simulink model "HybridBus_BEVModel"  (R2025a)
settings: Solver=FixedStepDiscrete  StartTime=0.0  StopTime=Input.Route.Time_s(end)  FixedStep=model_sample_time_s  RelTol=1e-3
InitFcn:
  | assign_hybrid_bus_model_workspace;
undefined symbols (not defined in the file): air_density_kg_m3, auxiliary_base_power_kw, auxiliary_override, battery1_charge_efficiency, battery1_discharge_efficiency, battery1_initial_energy_kwh, battery1_max_charge_kw, battery1_max_discharge_kw, battery1_max_energy_kwh, battery1_min_energy_kwh, battery1_usable_energy_kwh, battery2_charge_efficiency, battery2_discharge_efficiency, battery2_initial_energy_kwh, battery2_max_charge_kw, battery2_max_discharge_kw, battery2_max_energy_kwh, battery2_min_energy_kwh, battery2_usable_energy_kwh, BEVUseTwoBatteries, DiscIntNeverNeededParam, drag_coefficient, electricity_price_per_kWh, final_drive_motoring_efficiency, final_drive_ratio, final_drive_regen_efficiency, frontal_area_m2, fuel_price_per_L, gravity_m_s2, grid_charge_efficiency, model_sample_time_s, motor_max_speed_rpm, motor_motoring_efficiency, motor_regen_efficiency, motor_regen_limit_kw, motor_traction_limit_kw, rolling_coefficient, tyre_radius_m, vehicle_mass_kg
settings Model: Creator=Karuna  LastModifiedBy=Karuna
settings DataIOCC: SaveOutput=off  SignalLogging=off

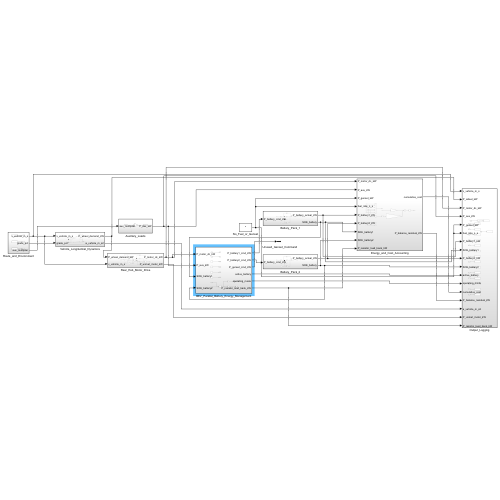
[thumbnail: Simulink's stored preview of the top-level diagram]
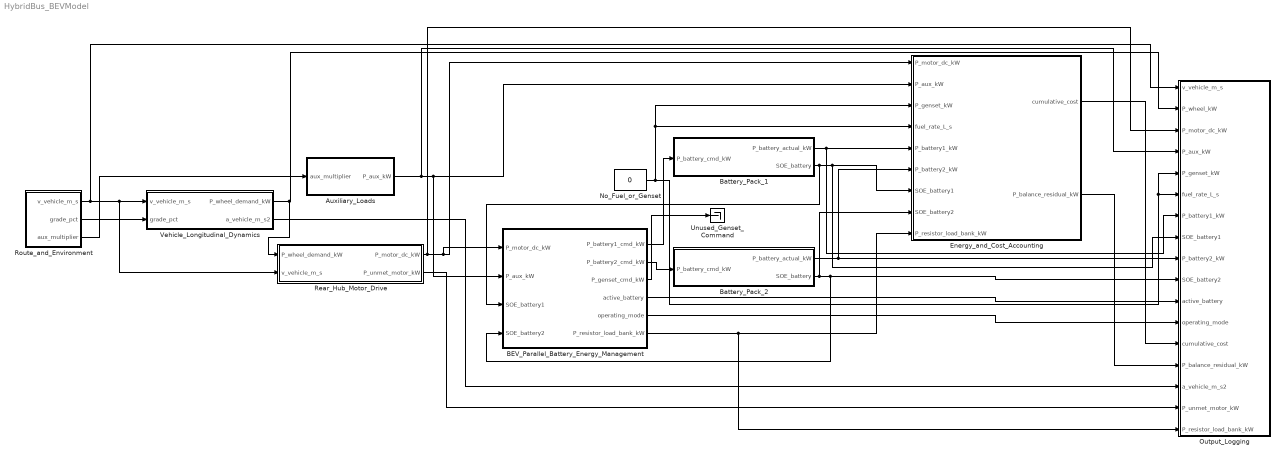
== system HybridBus_BEVModel ==
  Auxiliary_Loads : Subsystem
  BEV_Parallel_Battery_Energy_Management : Subsystem
  Battery_Pack_1 : Subsystem
  Battery_Pack_2 : Subsystem
  Energy_and_Cost_Accounting : Subsystem
  No_Fuel_or_Genset : Constant  Value=0
  Output_Logging : Subsystem
  Rear_Hub_Motor_Drive : Subsystem
  Route_and_Environment : Subsystem
  Unused_Genset_Command : Terminator
  Vehicle_Longitudinal_Dynamics : Subsystem
  wires:
  Route_and_Environment/2(grade_pct) -> Vehicle_Longitudinal_Dynamics/2(grade_pct)
  No_Fuel_or_Genset/1 -> Output_Logging/6(fuel_rate_L_s), Output_Logging/5(P_genset_kW), Energy_and_Cost_Accounting/4(fuel_rate_L_s), Energy_and_Cost_Accounting/3(P_genset_kW)
  Energy_and_Cost_Accounting/2(P_balance_residual_kW) -> Output_Logging/14(P_balance_residual_kW)
  Energy_and_Cost_Accounting/1(cumulative_cost) -> Output_Logging/13(cumulative_cost)
  Battery_Pack_2/1(P_battery_actual_kW) -> Energy_and_Cost_Accounting/6(P_battery2_kW), Output_Logging/9(P_battery2_kW)
  Battery_Pack_1/1(P_battery_actual_kW) -> Energy_and_Cost_Accounting/5(P_battery1_kW), Output_Logging/7(P_battery1_kW)
  Rear_Hub_Motor_Drive/2(P_unmet_motor_kW) -> Output_Logging/16(P_unmet_motor_kW)
  Vehicle_Longitudinal_Dynamics/2(a_vehicle_m_s2) -> Output_Logging/15(a_vehicle_m_s2)
  Vehicle_Longitudinal_Dynamics/1(P_wheel_demand_kW) -> Output_Logging/2(P_wheel_kW), Rear_Hub_Motor_Drive/1(P_wheel_demand_kW)
  Route_and_Environment/1(v_vehicle_m_s) -> Vehicle_Longitudinal_Dynamics/1(v_vehicle_m_s), Rear_Hub_Motor_Drive/2(v_vehicle_m_s), Output_Logging/1(v_vehicle_m_s)
  Route_and_Environment/3(aux_multiplier) -> Auxiliary_Loads/1(aux_multiplier)
  BEV_Parallel_Battery_Energy_Management/3(P_genset_cmd_kW) -> Unused_Genset_Command/1
  Battery_Pack_2/2(SOE_battery) -> Output_Logging/10(SOE_battery2), BEV_Parallel_Battery_Energy_Management/4(SOE_battery2), Energy_and_Cost_Accounting/8(SOE_battery2)
  Auxiliary_Loads/1(P_aux_kW) -> Energy_and_Cost_Accounting/2(P_aux_kW), BEV_Parallel_Battery_Energy_Management/2(P_aux_kW), Output_Logging/4(P_aux_kW)
  Rear_Hub_Motor_Drive/1(P_motor_dc_kW) -> Energy_and_Cost_Accounting/1(P_motor_dc_kW), BEV_Parallel_Battery_Energy_Management/1(P_motor_dc_kW), Output_Logging/3(P_motor_dc_kW)
  Battery_Pack_1/2(SOE_battery) -> Energy_and_Cost_Accounting/7(SOE_battery1), Output_Logging/8(SOE_battery1), BEV_Parallel_Battery_Energy_Management/3(SOE_battery1)
  BEV_Parallel_Battery_Energy_Management/1(P_battery1_cmd_kW) -> Battery_Pack_1/1(P_battery_cmd_kW)
  BEV_Parallel_Battery_Energy_Management/2(P_battery2_cmd_kW) -> Battery_Pack_2/1(P_battery_cmd_kW)
  BEV_Parallel_Battery_Energy_Management/4(active_battery) -> Output_Logging/11(active_battery)
  BEV_Parallel_Battery_Energy_Management/5(operating_mode) -> Output_Logging/12(operating_mode)
  BEV_Parallel_Battery_Energy_Management/6(P_resistor_load_bank_kW) -> Energy_and_Cost_Accounting/9(P_resistor_load_bank_kW), Output_Logging/17(P_resistor_load_bank_kW)

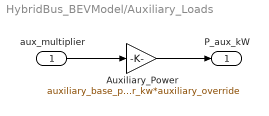
== system HybridBus_BEVModel/Auxiliary_Loads ==
  aux_multiplier : Inport
  Auxiliary_Power : Gain  Gain=auxiliary_base_power_kw*auxiliary_override
  P_aux_kW : Outport
  wires:
  Auxiliary_Power/1 -> P_aux_kW/1
  aux_multiplier/1 -> Auxiliary_Power/1

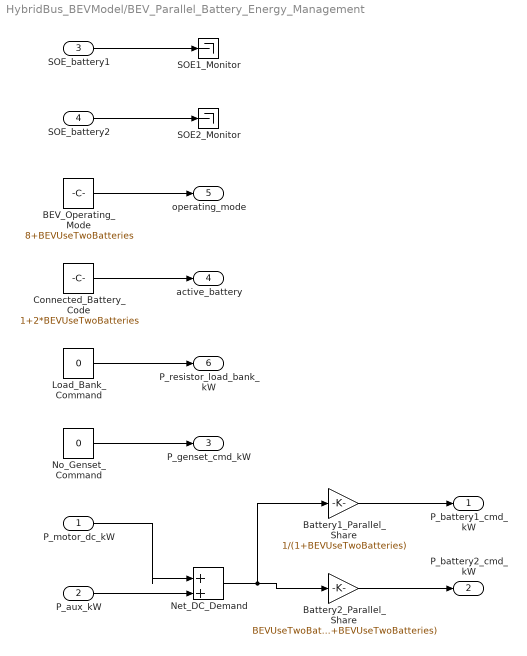
== system HybridBus_BEVModel/BEV_Parallel_Battery_Energy_Management ==
  P_motor_dc_kW : Inport
  P_aux_kW : Inport  Port=2
  SOE_battery1 : Inport  Port=3
  SOE_battery2 : Inport  Port=4
  BEV_Operating_Mode : Constant  Value=8+BEVUseTwoBatteries
  Battery1_Parallel_Share : Gain  Gain=1/(1+BEVUseTwoBatteries)
  Battery2_Parallel_Share : Gain  Gain=BEVUseTwoBatteries/(1+BEVUseTwoBatteries)
  Connected_Battery_Code : Constant  Value=1+2*BEVUseTwoBatteries
  Load_Bank_Command : Constant  Value=0
  Net_DC_Demand : Sum  Inputs=|++
  No_Genset_Command : Constant  Value=0
  SOE1_Monitor : Terminator
  SOE2_Monitor : Terminator
  P_battery1_cmd_kW : Outport
  P_battery2_cmd_kW : Outport  Port=2
  P_genset_cmd_kW : Outport  Port=3
  active_battery : Outport  Port=4
  operating_mode : Outport  Port=5
  P_resistor_load_bank_kW : Outport  Port=6
  wires:
  SOE_battery2/1 -> SOE2_Monitor/1
  SOE_battery1/1 -> SOE1_Monitor/1
  Load_Bank_Command/1 -> P_resistor_load_bank_kW/1
  BEV_Operating_Mode/1 -> operating_mode/1
  Connected_Battery_Code/1 -> active_battery/1
  No_Genset_Command/1 -> P_genset_cmd_kW/1
  Battery2_Parallel_Share/1 -> P_battery2_cmd_kW/1
  Battery1_Parallel_Share/1 -> P_battery1_cmd_kW/1
  Net_DC_Demand/1 -> Battery1_Parallel_Share/1, Battery2_Parallel_Share/1
  P_aux_kW/1 -> Net_DC_Demand/2
  P_motor_dc_kW/1 -> Net_DC_Demand/1

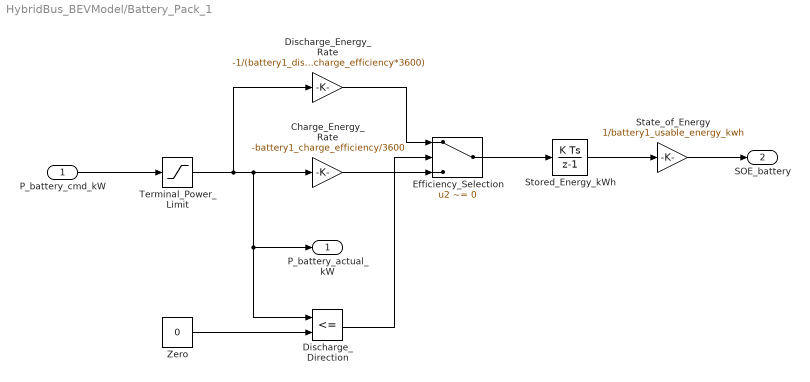
== system HybridBus_BEVModel/Battery_Pack_1 ==
  P_battery_cmd_kW : Inport
  Charge_Energy_Rate : Gain  Gain=-battery1_charge_efficiency/3600
  Discharge_Direction : RelationalOperator  Operator=<=  OutDataTypeStr=boolean  RndMeth=Simplest  InputSameDT=off
  Discharge_Energy_Rate : Gain  Gain=-1/(battery1_discharge_efficiency*3600)
  Efficiency_Selection : Switch  Criteria=u2 ~= 0  SaturateOnIntegerOverflow=off  InputSameDT=off
  State_of_Energy : Gain  Gain=1/battery1_usable_energy_kwh
  Stored_Energy_kWh : DiscreteIntegrator  InitialCondition=battery1_initial_energy_kwh  SampleTime=model_sample_time_s  LimitOutput=on  UpperSaturationLimit=battery1_max_energy_kwh  LowerSaturationLimit=battery1_min_energy_kwh  ICPrevOutput=DiscIntNeverNeededParam  ICPrevScaledInput=DiscIntNeverNeededParam
  Terminal_Power_Limit : Saturate  UpperLimit=battery1_max_discharge_kw  LowerLimit=-battery1_max_charge_kw
  Zero : Constant  Value=0
  P_battery_actual_kW : Outport
  SOE_battery : Outport  Port=2
  wires:
  State_of_Energy/1 -> SOE_battery/1
  Stored_Energy_kWh/1 -> State_of_Energy/1
  Efficiency_Selection/1 -> Stored_Energy_kWh/1
  Charge_Energy_Rate/1 -> Efficiency_Selection/3
  Discharge_Direction/1 -> Efficiency_Selection/2
  Discharge_Energy_Rate/1 -> Efficiency_Selection/1
  Zero/1 -> Discharge_Direction/2
  Terminal_Power_Limit/1 -> P_battery_actual_kW/1, Discharge_Direction/1, Charge_Energy_Rate/1, Discharge_Energy_Rate/1
  P_battery_cmd_kW/1 -> Terminal_Power_Limit/1

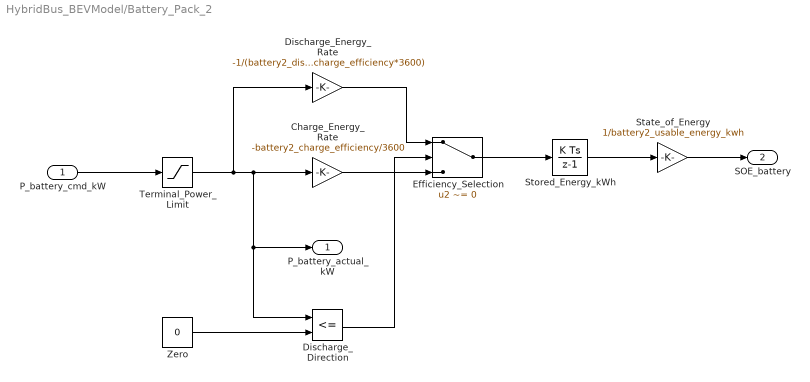
== system HybridBus_BEVModel/Battery_Pack_2 ==
  P_battery_cmd_kW : Inport
  Charge_Energy_Rate : Gain  Gain=-battery2_charge_efficiency/3600
  Discharge_Direction : RelationalOperator  Operator=<=  OutDataTypeStr=boolean  RndMeth=Simplest  InputSameDT=off
  Discharge_Energy_Rate : Gain  Gain=-1/(battery2_discharge_efficiency*3600)
  Efficiency_Selection : Switch  Criteria=u2 ~= 0  SaturateOnIntegerOverflow=off  InputSameDT=off
  State_of_Energy : Gain  Gain=1/battery2_usable_energy_kwh
  Stored_Energy_kWh : DiscreteIntegrator  InitialCondition=battery2_initial_energy_kwh  SampleTime=model_sample_time_s  LimitOutput=on  UpperSaturationLimit=battery2_max_energy_kwh  LowerSaturationLimit=battery2_min_energy_kwh  ICPrevOutput=DiscIntNeverNeededParam  ICPrevScaledInput=DiscIntNeverNeededParam
  Terminal_Power_Limit : Saturate  UpperLimit=battery2_max_discharge_kw  LowerLimit=-battery2_max_charge_kw
  Zero : Constant  Value=0
  P_battery_actual_kW : Outport
  SOE_battery : Outport  Port=2
  wires:
  State_of_Energy/1 -> SOE_battery/1
  Stored_Energy_kWh/1 -> State_of_Energy/1
  Efficiency_Selection/1 -> Stored_Energy_kWh/1
  Charge_Energy_Rate/1 -> Efficiency_Selection/3
  Discharge_Direction/1 -> Efficiency_Selection/2
  Discharge_Energy_Rate/1 -> Efficiency_Selection/1
  Zero/1 -> Discharge_Direction/2
  Terminal_Power_Limit/1 -> P_battery_actual_kW/1, Discharge_Direction/1, Charge_Energy_Rate/1, Discharge_Energy_Rate/1
  P_battery_cmd_kW/1 -> Terminal_Power_Limit/1

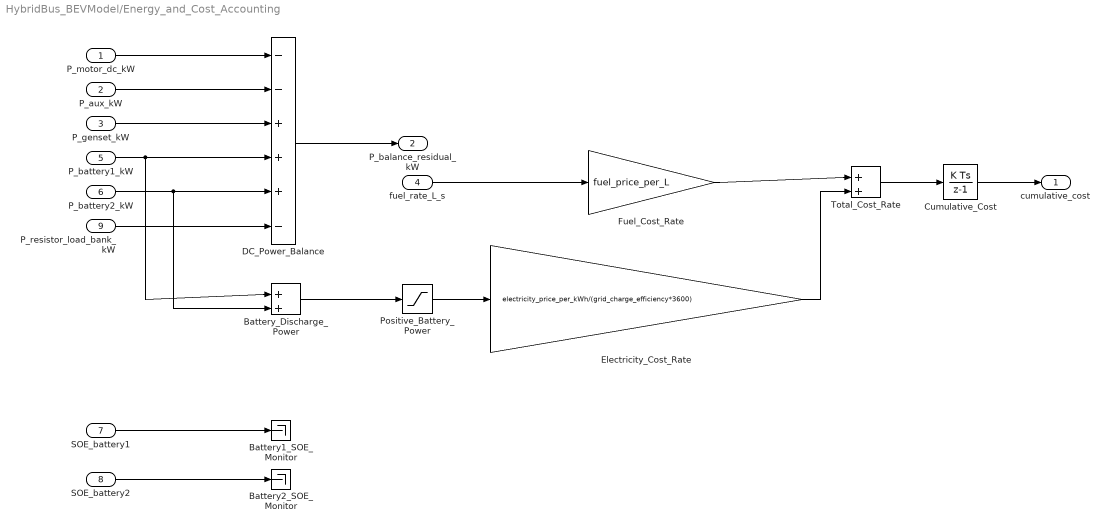
== system HybridBus_BEVModel/Energy_and_Cost_Accounting ==
  P_motor_dc_kW : Inport
  P_aux_kW : Inport  Port=2
  P_genset_kW : Inport  Port=3
  fuel_rate_L_s : Inport  Port=4
  P_battery1_kW : Inport  Port=5
  P_battery2_kW : Inport  Port=6
  SOE_battery1 : Inport  Port=7
  SOE_battery2 : Inport  Port=8
  P_resistor_load_bank_kW : Inport  Port=9
  Battery1_SOE_Monitor : Terminator
  Battery2_SOE_Monitor : Terminator
  Battery_Discharge_Power : Sum  Inputs=|++
  Cumulative_Cost : DiscreteIntegrator  SampleTime=model_sample_time_s  ICPrevOutput=DiscIntNeverNeededParam  ICPrevScaledInput=DiscIntNeverNeededParam
  DC_Power_Balance : Sum  Inputs=--+++-
  Electricity_Cost_Rate : Gain  Gain=electricity_price_per_kWh/(grid_charge_efficiency*3600)
  Fuel_Cost_Rate : Gain  Gain=fuel_price_per_L
  Positive_Battery_Power : Saturate  UpperLimit=inf  LowerLimit=0
  Total_Cost_Rate : Sum  Inputs=|++
  cumulative_cost : Outport
  P_balance_residual_kW : Outport  Port=2
  wires:
  fuel_rate_L_s/1 -> Fuel_Cost_Rate/1
  P_aux_kW/1 -> DC_Power_Balance/2
  P_battery2_kW/1 -> Battery_Discharge_Power/2, DC_Power_Balance/5
  P_motor_dc_kW/1 -> DC_Power_Balance/1
  P_genset_kW/1 -> DC_Power_Balance/3
  P_battery1_kW/1 -> Battery_Discharge_Power/1, DC_Power_Balance/4
  SOE_battery2/1 -> Battery2_SOE_Monitor/1
  Battery_Discharge_Power/1 -> Positive_Battery_Power/1
  P_resistor_load_bank_kW/1 -> DC_Power_Balance/6
  SOE_battery1/1 -> Battery1_SOE_Monitor/1
  Cumulative_Cost/1 -> cumulative_cost/1
  DC_Power_Balance/1 -> P_balance_residual_kW/1
  Total_Cost_Rate/1 -> Cumulative_Cost/1
  Positive_Battery_Power/1 -> Electricity_Cost_Rate/1
  Fuel_Cost_Rate/1 -> Total_Cost_Rate/1
  Electricity_Cost_Rate/1 -> Total_Cost_Rate/2

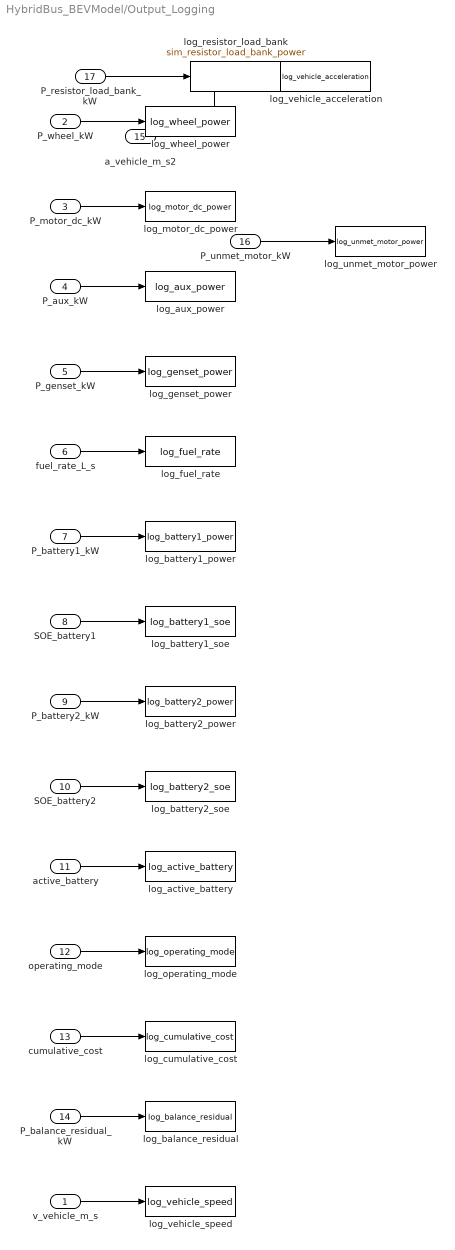
== system HybridBus_BEVModel/Output_Logging ==
  v_vehicle_m_s : Inport
  P_wheel_kW : Inport  Port=2
  P_motor_dc_kW : Inport  Port=3
  P_aux_kW : Inport  Port=4
  P_genset_kW : Inport  Port=5
  fuel_rate_L_s : Inport  Port=6
  P_battery1_kW : Inport  Port=7
  SOE_battery1 : Inport  Port=8
  P_battery2_kW : Inport  Port=9
  SOE_battery2 : Inport  Port=10
  active_battery : Inport  Port=11
  operating_mode : Inport  Port=12
  cumulative_cost : Inport  Port=13
  P_balance_residual_kW : Inport  Port=14
  a_vehicle_m_s2 : Inport  Port=15
  P_unmet_motor_kW : Inport  Port=16
  P_resistor_load_bank_kW : Inport  Port=17
  log_active_battery : ToWorkspace  VariableName=log_active_battery  SaveFormat=Timeseries  SampleTime=-1
  log_aux_power : ToWorkspace  VariableName=log_aux_power  SaveFormat=Timeseries  SampleTime=-1
  log_balance_residual : ToWorkspace  VariableName=log_balance_residual  SaveFormat=Timeseries  SampleTime=-1
  log_battery1_power : ToWorkspace  VariableName=log_battery1_power  SaveFormat=Timeseries  SampleTime=-1
  log_battery1_soe : ToWorkspace  VariableName=log_battery1_soe  SaveFormat=Timeseries  SampleTime=-1
  log_battery2_power : ToWorkspace  VariableName=log_battery2_power  SaveFormat=Timeseries  SampleTime=-1
  log_battery2_soe : ToWorkspace  VariableName=log_battery2_soe  SaveFormat=Timeseries  SampleTime=-1
  log_cumulative_cost : ToWorkspace  VariableName=log_cumulative_cost  SaveFormat=Timeseries  SampleTime=-1
  log_fuel_rate : ToWorkspace  VariableName=log_fuel_rate  SaveFormat=Timeseries  SampleTime=-1
  log_genset_power : ToWorkspace  VariableName=log_genset_power  SaveFormat=Timeseries  SampleTime=-1
  log_motor_dc_power : ToWorkspace  VariableName=log_motor_dc_power  SaveFormat=Timeseries  SampleTime=-1
  log_operating_mode : ToWorkspace  VariableName=log_operating_mode  SaveFormat=Timeseries  SampleTime=-1
  log_resistor_load_bank : ToWorkspace  VariableName=sim_resistor_load_bank_power  SampleTime=-1
  log_unmet_motor_power : ToWorkspace  VariableName=log_unmet_motor_power  SaveFormat=Timeseries  SampleTime=-1
  log_vehicle_acceleration : ToWorkspace  VariableName=log_vehicle_acceleration  SaveFormat=Timeseries  SampleTime=-1
  log_vehicle_speed : ToWorkspace  VariableName=log_vehicle_speed  SaveFormat=Timeseries  SampleTime=-1
  log_wheel_power : ToWorkspace  VariableName=log_wheel_power  SaveFormat=Timeseries  SampleTime=-1
  wires:
  P_balance_residual_kW/1 -> log_balance_residual/1
  cumulative_cost/1 -> log_cumulative_cost/1
  operating_mode/1 -> log_operating_mode/1
  active_battery/1 -> log_active_battery/1
  SOE_battery2/1 -> log_battery2_soe/1
  P_battery2_kW/1 -> log_battery2_power/1
  SOE_battery1/1 -> log_battery1_soe/1
  P_battery1_kW/1 -> log_battery1_power/1
  fuel_rate_L_s/1 -> log_fuel_rate/1
  P_genset_kW/1 -> log_genset_power/1
  P_aux_kW/1 -> log_aux_power/1
  P_motor_dc_kW/1 -> log_motor_dc_power/1
  P_wheel_kW/1 -> log_wheel_power/1
  v_vehicle_m_s/1 -> log_vehicle_speed/1
  P_unmet_motor_kW/1 -> log_unmet_motor_power/1
  P_resistor_load_bank_kW/1 -> log_resistor_load_bank/1
  a_vehicle_m_s2/1 -> log_vehicle_acceleration/1

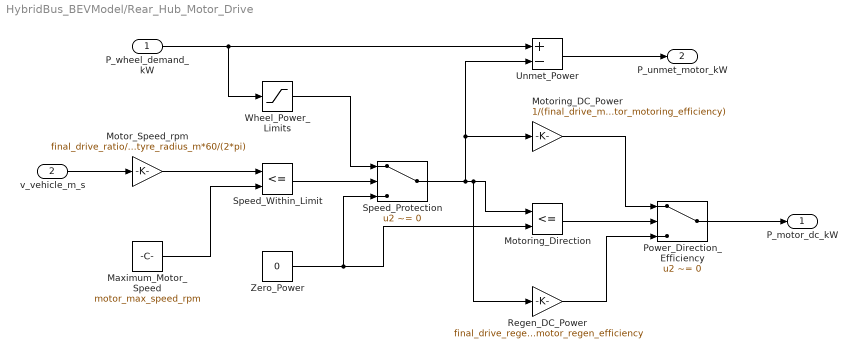
== system HybridBus_BEVModel/Rear_Hub_Motor_Drive ==
  P_wheel_demand_kW : Inport
  v_vehicle_m_s : Inport  Port=2
  Maximum_Motor_Speed : Constant  Value=motor_max_speed_rpm
  Motor_Speed_rpm : Gain  Gain=final_drive_ratio/tyre_radius_m*60/(2*pi)
  Motoring_DC_Power : Gain  Gain=1/(final_drive_motoring_efficiency*motor_motoring_efficiency)
  Motoring_Direction : RelationalOperator  Operator=<=  OutDataTypeStr=boolean  RndMeth=Simplest  InputSameDT=off
  Power_Direction_Efficiency : Switch  Criteria=u2 ~= 0  SaturateOnIntegerOverflow=off  InputSameDT=off
  Regen_DC_Power : Gain  Gain=final_drive_regen_efficiency*motor_regen_efficiency
  Speed_Protection : Switch  Criteria=u2 ~= 0  SaturateOnIntegerOverflow=off  InputSameDT=off
  Speed_Within_Limit : RelationalOperator  Operator=<=  OutDataTypeStr=boolean  RndMeth=Simplest  InputSameDT=off
  Unmet_Power : Sum  Inputs=+-
  Wheel_Power_Limits : Saturate  UpperLimit=motor_traction_limit_kw  LowerLimit=-motor_regen_limit_kw
  Zero_Power : Constant  Value=0
  P_motor_dc_kW : Outport
  P_unmet_motor_kW : Outport  Port=2
  wires:
  Unmet_Power/1 -> P_unmet_motor_kW/1
  Power_Direction_Efficiency/1 -> P_motor_dc_kW/1
  Regen_DC_Power/1 -> Power_Direction_Efficiency/3
  Motoring_Direction/1 -> Power_Direction_Efficiency/2
  Motoring_DC_Power/1 -> Power_Direction_Efficiency/1
  Speed_Protection/1 -> Regen_DC_Power/1, Motoring_Direction/1, Motoring_DC_Power/1, Unmet_Power/2
  Zero_Power/1 -> Speed_Protection/3, Motoring_Direction/2
  Speed_Within_Limit/1 -> Speed_Protection/2
  Wheel_Power_Limits/1 -> Speed_Protection/1
  Maximum_Motor_Speed/1 -> Speed_Within_Limit/2
  Motor_Speed_rpm/1 -> Speed_Within_Limit/1
  v_vehicle_m_s/1 -> Motor_Speed_rpm/1
  P_wheel_demand_kW/1 -> Unmet_Power/1, Wheel_Power_Limits/1

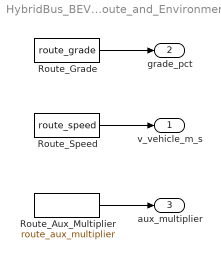
== system HybridBus_BEVModel/Route_and_Environment ==
  Route_Aux_Multiplier : FromWorkspace  VariableName=route_aux_multiplier
  Route_Grade : FromWorkspace  VariableName=route_grade
  Route_Speed : FromWorkspace  VariableName=route_speed
  v_vehicle_m_s : Outport
  grade_pct : Outport  Port=2
  aux_multiplier : Outport  Port=3
  wires:
  Route_Aux_Multiplier/1 -> aux_multiplier/1
  Route_Grade/1 -> grade_pct/1
  Route_Speed/1 -> v_vehicle_m_s/1

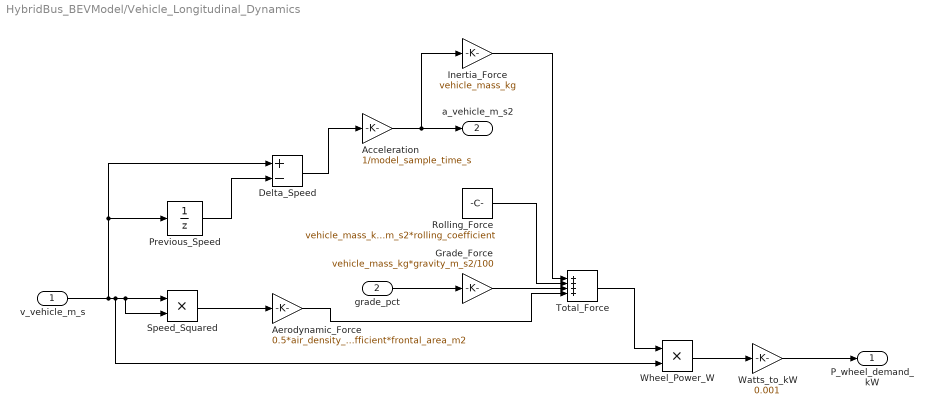
== system HybridBus_BEVModel/Vehicle_Longitudinal_Dynamics ==
  v_vehicle_m_s : Inport
  grade_pct : Inport  Port=2
  Acceleration : Gain  Gain=1/model_sample_time_s
  Aerodynamic_Force : Gain  Gain=0.5*air_density_kg_m3*drag_coefficient*frontal_area_m2
  Delta_Speed : Sum  Inputs=+-
  Grade_Force : Gain  Gain=vehicle_mass_kg*gravity_m_s2/100
  Inertia_Force : Gain  Gain=vehicle_mass_kg
  Previous_Speed : UnitDelay  SampleTime=model_sample_time_s  HasFrameUpgradeWarning=on
  Rolling_Force : Constant  Value=vehicle_mass_kg*gravity_m_s2*rolling_coefficient
  Speed_Squared : Product  Inputs=**
  Total_Force : Sum  Inputs=++++
  Watts_to_kW : Gain  Gain=0.001
  Wheel_Power_W : Product  Inputs=**
  P_wheel_demand_kW : Outport
  a_vehicle_m_s2 : Outport  Port=2
  wires:
  Watts_to_kW/1 -> P_wheel_demand_kW/1
  Wheel_Power_W/1 -> Watts_to_kW/1
  Total_Force/1 -> Wheel_Power_W/1
  Aerodynamic_Force/1 -> Total_Force/4
  Grade_Force/1 -> Total_Force/3
  Rolling_Force/1 -> Total_Force/2
  Inertia_Force/1 -> Total_Force/1
  Speed_Squared/1 -> Aerodynamic_Force/1
  grade_pct/1 -> Grade_Force/1
  Acceleration/1 -> a_vehicle_m_s2/1, Inertia_Force/1
  Delta_Speed/1 -> Acceleration/1
  Previous_Speed/1 -> Delta_Speed/2
  v_vehicle_m_s/1 -> Speed_Squared/1, Speed_Squared/2, Wheel_Power_W/2, Previous_Speed/1, Delta_Speed/1
